simulink library "Ampere_Library"  (R2022b)
settings: Solver=FixedStepDiscrete  StartTime=0  StopTime=10.0  RelTol=1e-3  EnableMultiTasking=on
undefined symbols (not defined in the file or in its folder): A_INST_double, Dem_EventStatusType, ECU_AMBIENT_TEMPERATURE, SET_ECU_AMBIENT_TEMPERATURE, SlDemoSign, Std_ReturnType
libraries: simulink x13
(part 5 of 10)

== system Ampere_Library/User_Defined_Libraries/Signal_Routing ==
  note: Specific
  note: Invalid Values
  note: Signal Routing
  note: Obsolete
  A_DataTypeDuplicate : Subsystem  Tag=[LIB]  mask(A_DataTypeDuplicate){NoIn=3}
      mask prompts: NoIn "No Of Inputs"
      mask help:
      | ****************************************************************************
      | DO NOT USE THIS BLOCK ANYMORE.
      | Use the native "Same DT" block in the section MBD_Base_Blocks / Simulink / Signal_Attributes
      |
      | ****************************************************************************
      |
      | This block forces all inputs to have the exact same data type. The user shall set the number of the inputs in the mask parameter
      mask init:
      | % This code add/delete inports and matching lines to connect to the mux
      | % block.
      | 
      | % Number of inputs to have
      | f = str2num(get_param(gcb, 'NoIn'));
      | % Get all existing inports
      | d1 = find_system(gcb,'LookUnderMasks','all','Followlinks','on','BlockType','Inport');
      | 
      | % Update the mux block
      | set_param([gcb '/Mux'],'Inputs',num2str(f));
      | 
      | % Update content if new value different from number of existing inports
      | if f ~= length(d1)
      |     % Delete all existing inports and matching lines
      |     for i = 1:length(d1)
      |         hanblk = get_param(d1{i},'handle');
      |         blkDet = get(hanblk);
      |         pos = blkDet.PortConnectivity(1).Position;
      |         delete_line(gcb,pos);
      |         delete_block(d1{i});
      |     end
      |     
      |     % Add new ports and lintes
      |     for i = 1:f
      |         b = i*50;
      |         a = 150;
      |         append = num2str(i);
      |         append = strcat('/In',append);
      |     	PortName = strcat(gcb,append);
      |         add_block('built-in/Inport',PortName,'Position',[a-60 b-5 a-40 b+8],'FontName','Arial','FontSize',12);
      |         set_param(PortName,'ShowName','On')
      |         set_param(PortName,'Backgroundcolor','green');
      |         new_line = add_line(gcb,['In' num2str(i) '/1'],['Mux/' num2str(i)],'Autorouting','On');
      |         set(new_line,'FontName','Arial');
      |         set(new_line,'FontSize','12');
      |     end
      | end
      settings: AttributesFormatString="%<MaskType>  \\n No Of Inputs = %<NoIn>"
      mask Display:
      | %% Display info on the icon
      | fprintf('Same\nDT')
  A_DefaultValueSwitch : Subsystem  Tag=[LIB]  mask(A_DefaultValueSwitch){DefaultValue=15.1, InvalidValue=2.1, tolerance=double tol - eps('double'), user_tol=0, SaturateOnOverflow=off}
      mask prompts: DefaultValue "Default Value"; InvalidValue "Invalid Value"; tolerance "Tolerance for Invalid Value"; user_tol "User Defined Tolerance"; SaturateOnOverflow "Saturate on integer overflow"
      mask help:
      | This block outputs default value, in case of a invalid input. Otherwise output follows input.
      |
      | When parameter 'Invalid Value' and the input "U" is equal, then the output "Y" is equal to the 'Default Value' parameter. Otherwise the output "Y" is equal to the input "U".
      mask init:
      | %% Compute Tolerance
      | switch tolerance
      |     case 1
      |         tol = eps('double');
      |     case 2
      |         tol = eps('single');
      |     case 3
      |         tol = 0;
      |     case 4
      |         tol = user_tol;
      | end
      | 
      | %% Create the infos to display below the block depending of the Mask Options
      | % Always display MaskType
      | Attrib = '%<MaskType>';
      | % Conditionnally adding Tolerance
      | if strcmp(get_param(gcb,'tolerance'),'User Defined tol')
      |     Attrib = [Attrib '\nTol = %<user_tol>'];
      | end
      | % Conditionnally adding Sat
      | if strcmp(get_param(gcb,'SaturateOnOverflow'),'on')
      |     Attrib = [Attrib '\nSAT = on'];
      | end
      | % Update the display
      | set_param(gcb,'AttributesFormatString',Attrib);
      settings: AttributesFormatString=%<MaskType>
      mask TypeOptions tolerance: double tol - eps('double') | single tol - eps('single') | Absolute Zero tol | User Defined tol
      mask Callback tolerance:
      | %% Make visible or not the Tolerance (update 2nd element of MaskVisibilities)
      | MaskVisibilities = get_param(gcb,'MaskVisibilities');
      | if strcmp(get_param(gcb,'tolerance'),'User Defined tol')
      |     MaskVisibilities{4} = 'on';
      | else
      |     MaskVisibilities{4} = 'off';
      | end
      | set_param(gcb,'MaskVisibilities',MaskVisibilities);
      mask TypeOptions SaturateOnOverflow: Add/SaturateOnIntegerOverflow | Add1/SaturateOnIntegerOverflow | Switch2/SaturateOnIntegerOverflow
      mask Display:
      | %% Display info on the icon
      | fprintf('Default Val = %s\nInvalid Val = %s', get_param(gcb,'DefaultValue'),get_param(gcb,'InvalidValue'));
  A_ExtDefaultValueSw : Subsystem  Tag=[LIB]  mask(A_ExtDefaultValueSw){InvalidValue=0, tolerance=Absolute Zero tol, user_tol=2.5, SATonIntegerOverflow=off}
      mask prompts: InvalidValue "Invalid Value"; tolerance "Tolerance for Invalid Value"; user_tol "User Defined Tolerance"; SATonIntegerOverflow "Saturate on integer overflow"
      mask help:
      | When parameter 'Invalid Value' and input "Inp2" are equal then, the output "Y"  is equal to the input "Inp1". Otherwise the output "Y" is equal to the input "In2".
      | Note:
      | 1) If tolerance value is given for double/single data type, then the parameter "Invalid value" should be given within the range as given below
      | MAX value = ('double/single') MAX-Tolerance
      | MIN value = ('double/single') MIN+Tolerance
      mask init:
      | %% Compute Tolerance
      | switch tolerance
      |     case 1
      |         tol = eps('double');
      |     case 2
      |         tol = eps('single');
      |     case 3
      |         tol = 0;
      |     case 4
      |         tol = user_tol;
      | end
      | 
      | %% Create the infos to display below the block depending of the Mask Options
      | % Always display MaskType
      | Attrib = '%<MaskType>\nInvalidVal = %<InvalidValue>';
      | % Conditionnally adding Tolerance
      | if strcmp(get_param(gcb,'tolerance'),'User Defined tol')
      |     Attrib = [Attrib '\nTol = %<user_tol>'];
      | end
      | % Conditionnally adding Sat
      | if strcmp(get_param(gcb,'SATonIntegerOverflow'),'on')
      |     Attrib = [Attrib '\nSAT = on'];
      | end
      | % Update the display
      | set_param(gcb,'AttributesFormatString',Attrib);
      settings: AttributesFormatString=%<MaskType>\nInvalidVal = %<InvalidValue>
      mask TypeOptions tolerance: double tol - eps('double') | single tol - eps('single') | Absolute Zero tol | User Defined tol
      mask Callback tolerance:
      | %% Make visible or not the Tolerance (update 3nd element of MaskVisibilities)
      | MaskVisibilities = get_param(gcb,'MaskVisibilities');
      | if strcmp(get_param(gcb,'tolerance'),'User Defined tol')
      |     MaskVisibilities{3} = 'on';
      | else
      |     MaskVisibilities{3} = 'off';
      | end
      | set_param(gcb,'MaskVisibilities',MaskVisibilities);
      mask TypeOptions SATonIntegerOverflow: Switch2/SaturateOnIntegerOverflow | Add/SaturateOnIntegerOverflow | Add1/SaturateOnIntegerOverflow
  A_ResolutionBlock : Subsystem  Tag=[LIB]  mask(A_ResolutionBlock){Resolution=1, SaturateOnOverflow=off, prod_OutDataTypeStr=double}
      mask prompts: Resolution "Signal resolution resizing"; SaturateOnOverflow "Saturate on integer overflow"; prod_OutDataTypeStr "Simulink:blkprm_prompts:OUTPUT_UNIFIEDDATATYPE"
      mask help:
      | This block converts input signal 'U' value into the value 'Y', with resolution specified by 'Signal resolution resizing' mask parameter.
      |
      | Conversion is done using following formula:
      |
      | Y = [ROUND ( U / Resolution )] * Resolution
      |
      | Note:
      | 1.  Input (U) Datatype of the block must be "DOUBLE".
      | 2. Output data type of the block has to be chosen by the user through "Output data type" mask parameter.
      mask init:
      | %% Internal Parameters
      | RF0 = 0;
      | RF1 = 1;
      | RF05 = 0.5;
      settings: AttributesFormatString=%<MaskType>
      mask TypeOptions SaturateOnOverflow: Product1/SaturateOnIntegerOverflow
      mask Callback SaturateOnOverflow:
      | %% Create the infos to display below the block depending of the Mask Options
      | % Always display MaskType
      | Attrib = '%<MaskType>';
      | % Conditionnally adding Sat
      | if strcmp(get_param(gcb,'SaturateOnOverflow'),'on')
      |     Attrib = [Attrib '\nSAT = on'];
      | end
      | % Update the display
      | set_param(gcb,'AttributesFormatString',Attrib);
      mask TypeOptions prod_OutDataTypeStr: Product1/OutDataTypeStr
      mask DialogControl prod_OutDataTypeStr Prompt: Output data type:
      mask Display:
      | %% Display info on the icon
      | fprintf('Resol :\n%s', get_param(gcb,'Resolution'));
  A_SlopeSwitch2Inputs : Subsystem  Tag=[LIB]  mask(A_SlopeSwitch2Inputs){st=0.1, SaturateOnIntegerOverflow=off}
      mask prompts: st "Sample Time used for calculation, should not be inherited (-1)."; SaturateOnIntegerOverflow "Simulink:blkprm_prompts:AllBlksSaturate"
      mask help:
      | This block is a Multi-Port Slope Switch.
      | Depending on the value of input Switch_Cmd (zero-based), the block outputs the corresponding input signal.
      | For Switch_Cmd = 0, Outis Inp0, for Switch_Cmd = 1, Out is Inp1, and so on...
      |
      | Nevertheless, for each switch between two input signals, a slope is activated from the first input signal to the second input signal.
      | The value of this slope is given by Pos_Slope if the input signal to reach is over the initial input signal and by Neg_Slope if the input signal to reach is under.
      | Pos_Slope and Neg_Slope are respectively the positive and negative slope parameters per second.
      |
      | The output Slope_On indicates if a transition is active (Slope_On at true) or not (Slope_On at false).
      |
      | In order to avoid the overflow, the maximum/ minimun range for the inputs Pos_Slope and Neg_Slope shall be choosen as:
      | max range(Pos_Slope) = ( max range(data type(In))- max(In))
      | min range(Neg_Slope) = ( min range(data type(Input)) - min(Input))
      |
      | Note:
      | 1. Data type for the outport "Out" will be same as "Inp0" or "Inp1" (Inp0 and Inp1 should be same data type)
      | 2. Data type for the outport "Slope_On" is always "boolean".
      mask init:
      | %% Internal Parameters
      | InitDelay = 0;
      | InitOut = 0;
      settings: AttributesFormatString=%<MaskType>
      mask TypeOptions SaturateOnIntegerOverflow: Multiport_Switch/SaturateOnIntegerOverflow | Slope_On_Block/Product/SaturateOnIntegerOverflow | Slope_On_Block/Product1/SaturateOnIntegerOverflow | Slope_On_Block/Sum/SaturateOnIntegerOverflow | Slope_On_Block/Sum1/SaturateOnIntegerOverflow | Slope_On_Block/Switch1/SaturateOnIntegerOverflow | Slope_On_Block/Switch2/SaturateOnIntegerOverflow | Slope_On_Block/Switch3/SaturateOnIntegerOverflow | Switch2/SaturateOnIntegerOverflow
      mask Callback SaturateOnIntegerOverflow:
      | %% Create the infos to display below the block depending of the Mask Options
      | % Always display MaskType
      | Attrib = '%<MaskType>';
      | % Conditionnally adding Sat
      | if strcmp(get_param(gcb,'SaturateOnIntegerOverflow'),'on')
      |     Attrib = [Attrib '\nSAT = on'];
      | end
      | % Update the display
      | set_param(gcb,'AttributesFormatString',Attrib);
      mask DialogControl SaturateOnIntegerOverflow Prompt: Saturate on integer overflow
      mask Display:
      | %% Display info on the icon
      | color('blue')
      | fprintf('Slope switch\n\n2 Inputs')
  A_TwoInDefltValSwitch : Subsystem  Tag=[LIB]  mask(A_TwoInDefltValSwitch){DefaultValue=15.1, InvalidValue=2.1, tolerance=double tol - eps('double'), user_tol=2.5, SATOnIntegerOverflow=off}
      mask prompts: DefaultValue "Default Value"; InvalidValue "Invalid Value"; tolerance "Tolerance for Invalid Value"; user_tol "User Defined Tolerance"; SATOnIntegerOverflow "Saturate on integer overflow"
      mask help: Compare the input2 'U2' with the invalid value ,if it is equal then the output 'Y' is Default value,otherwise the output is as same as input1 'U1'.
      mask init:
      | %% Compute Tolerance
      | switch tolerance
      |     case 1
      |         tol = eps('double');
      |     case 2
      |         tol = eps('single');
      |     case 3
      |         tol = 0;
      |     case 4
      |         tol = user_tol;
      | end
      | 
      | %% Create the infos to display below the block depending of the Mask Options
      | % Always display MaskType
      | Attrib = '%<MaskType>';
      | % Conditionnally adding Tolerance
      | if strcmp(get_param(gcb,'tolerance'),'User Defined tol')
      |     Attrib = [Attrib '\nTol = %<user_tol>'];
      | end
      | % Conditionnally adding Sat
      | if strcmp(get_param(gcb,'SATOnIntegerOverflow'),'on')
      |     Attrib = [Attrib '\nSAT = on'];
      | end
      | % Update the display
      | set_param(gcb,'AttributesFormatString',Attrib);
      settings: AttributesFormatString=%<MaskType>
      mask TypeOptions tolerance: double tol - eps('double') | single tol - eps('single') | Absolute Zero tol | User Defined tol
      mask Callback tolerance:
      | %% Make visible or not the Tolerance (update 2nd element of MaskVisibilities)
      | MaskVisibilities = get_param(gcb,'MaskVisibilities');
      | if strcmp(get_param(gcb,'tolerance'),'User Defined tol')
      |     MaskVisibilities{4} = 'on';
      | else
      |     MaskVisibilities{4} = 'off';
      | end
      | set_param(gcb,'MaskVisibilities',MaskVisibilities);
      mask TypeOptions SATOnIntegerOverflow: Switch2/SaturateOnIntegerOverflow | Add/SaturateOnIntegerOverflow | Add1/SaturateOnIntegerOverflow
      mask Display:
      | %% Display info on the icon
      | fprintf('Default Val = %s\nInvalid Val = %s', get_param(gcb,'DefaultValue'), get_param(gcb,'InvalidValue'));
  A_demux_fc : Subsystem  Tag=[LIB]  Description=This block is let for backwards compatibility. Function-call generator blocks are forbiddenby LB001 rule. Users shall modify their models if this block is used.  mask(A_demux_fc){}
      mask help:
      | ****************************************************************************
      | DO NOT USE THIS BLOCK ANYMORE.
      | This block is let for backwards compatibility. Function-call generator blocks are forbiddenby LB001 rule. Users shall modify their models if this block is used
      | ****************************************************************************
      |
      | A_demux_fc block shall be use before demuxing function call signal.
      settings: AttributesFormatString=%<MaskType>  RTWSystemCode=Inline

== system Ampere_Library/User_Defined_Libraries/Sources ==
  note: Sources
  A_ClockGen : Subsystem  Tag=[LIB]  mask(A_ClockGen){st=0.1, SaturateOnOverflow=off, const_OutDataTypeStr=double}
      mask prompts: st "Sample time is used in calculation, should not be inherited (-1)"; SaturateOnOverflow "Saturate on integer overflow"; const_OutDataTypeStr "Sample time Datatype"
      mask help:
      | This block outputs the simulation time, when it is kept inside the time based subsystem. The parameter "sample time" should be explicitly mentioned.
      | Inherit value '-1' is not allowed.
      |
      | Note: Datatype of the given Sample time has to be chosen by the user through "Sample time Datatype" mask parameter.
      mask init:
      | %% Internal Parameter
      | InitClock = 0;
      | 
      | %% Check Sample Time
      | if st < 0
      |     errordlg(['Error : Do not use inherited sample time -1 in ',gcb]);
      | end
      settings: AttributesFormatString=|
      | %<MaskType>
      | Sample Time = %<st>
      mask TypeOptions SaturateOnOverflow: Sum1/SaturateOnIntegerOverflow
      mask Callback SaturateOnOverflow:
      | % Display the SaturateOnOverflow parameter only when 'on'
      | if strcmp(get_param(gcb,'SaturateOnOverflow'),'on')
      |     set_param(gcb, 'AttributesFormatString', sprintf('%%<MaskType>\nSample Time = %%<st> \nSAT = on'));
      | else
      |     set_param(gcb, 'AttributesFormatString', sprintf('%%<MaskType>\nSample Time = %%<st> \n'));
      | end
      mask TypeOptions const_OutDataTypeStr: st/OutDataTypeStr
      mask Display:
      | %% Display info on the icon
      | fprintf('Digital\nclock');
  A_DownEdge_Event : Subsystem  Tag=[LIB]  mask(A_DownEdge_Event){sample_time=0.01, event_time=0.1, InternalDT=double}
      mask prompts: sample_time "Sample time for calculations"; event_time "Event production time"; InternalDT "Internal Calculations Data Type"
      mask help:
      | Down edge event  : Every Event_time
      |
      | The block produces a Down Edge Boolean output every period of time defined by:
      | Event production time: period of time between two Down Edge events.
      |
      | * This block shall not be used inside triggered/enabled subsystem
      mask init:
      | %% Check for Internal Calculations Data Type 
      | if strcmp(get_param(gcb, 'InternalDT'), 'double')
      |     imm_clear = double(0);
      |     imm = double(0.0001);
      |     sample_time = double(sample_time);
      |     event_time = double(event_time);
      | else
      |     imm_clear = single(0);
      |     imm = single(0.0001);
      |     sample_time = single(sample_time);
      |     event_time = single(event_time);
      | end
      settings: AttributesFormatString=|
      | %<MaskType>
      | Internal DT = %<InternalDT>
      mask Display:
      | %% Display info on the icon
      | fprintf('Sample Time = %s\nEvent Time = %s', get_param(gcb,'sample_time'),get_param(gcb,'event_time'));
  A_EnumConstant : Subsystem  Tag=[LIB]  mask{OutDataTypeStr=Enum: SlDemoSign, EnumVal=Positive}
      mask prompts: OutDataTypeStr "Output data type"; EnumVal "Value"
      mask help: This block is customized to display an enumerated value in a more compact way and avoid giant blocks that degrade the readibility.
      mask init:
      | %% Retrieve the enum name and its value in the mask
      | Type = regexprep(strrep(get(gcbh,'OutDataTypeStr'),' ',''),'Enum:','');
      | Value = strtrim(get(gcbh,'EnumVal'));
      | 
      | %% Compute the enumerated value to put in the constant block
      | Ecst = eval([Type  '.'  Value]);
      settings: AttributesFormatString=Enum: SlDemoSign
      mask Callback OutDataTypeStr:
      | %% Get the enum name
      | Type = get(gcbh,'OutDataTypeStr');
      | 
      | %% Get its enumeration values as a char array to then create the new value
      | % of MaskStyles properties to update the popupmenu in the mask
      | ListVal = char(string(enumeration(regexprep(strrep(Type,' ',''),'Enum:',''))));
      | NewList = [];
      | for i = 1:size(ListVal,1)
      |     NewList = [NewList ListVal(i,:) '|'];
      | end
      | NewList(end) = [];
      | 
      | %% Update MaskStyles with the new values for the popupmenu
      | MaskStyles = get(gcbh,'MaskStyles');
      | MaskStyles{2} = ['popup(' NewList ')'];
      | set(gcbh,'MaskStyles',MaskStyles);
      | 
      | %% Update display below the block
      | set(gcbh,'AttributesFormatString',get(gcbh,'OutDataTypeStr'));
      mask TypeOptions EnumVal: Positive | Zero     | Negative
      mask Display:
      | %% Display the enum below the block and the value on the subsystem
      | fprintf('%s',strtrim(get(gcbh,'EnumVal')));

== system Ampere_Library/User_Defined_Libraries/Timers_and_Counters ==
  note: Timers
  note: Counters
  note: Turn On/Off Delays
  note: Timers & Counters
  A_COUNTER : Subsystem  Tag=[LIB]  mask(A_COUNTER){mMAX=1byte, SaturateOnOverflow=off}
      mask prompts: mMAX "Max. count range :"; SaturateOnOverflow "Saturate on integer overflow"
      mask help:
      | When the input of the block ("start_flag") gets the value 1 (True), the output value ("count_value") will be incremented at each simulation step until reaching the maximum value fixed by user and then, maintain the limit value.
      |
      | When the input of the block ("start_flag") gets the value 0 (False), the output value ("count_value") will be set to '0'
      |
      |
      | Note
      | The input of the block shall be a Boolean
      mask init:
      | %% Internal Parameters
      | IncrVal = 1;
      | ClrVal = 0;
      | IC_zero = 0;
      | 
      | %% Compute the limit value depending of the number of bytes
      | mMAX = get_param(gcb,'mMAX');
      | nbByte = str2double(mMAX(1)); % first element is either 1/2/4
      | MavVal = 2^(nbByte * 8 ) - 1;
      | 
      | if nbByte == 1
      |     limit_value = uint8(MavVal);
      | elseif nbByte == 2
      |     limit_value = uint16(MavVal);
      | else % nbByte == 4
      |     limit_value = uint32(MavVal);
      | end
      settings: AttributesFormatString=%<MaskType>
      mask TypeOptions mMAX: 1byte | 2byte | 4byte
      mask TypeOptions SaturateOnOverflow: Min/SaturateOnIntegerOverflow | Sum1/SaturateOnIntegerOverflow | Switch1/SaturateOnIntegerOverflow
      mask Callback SaturateOnOverflow:
      | %% Create the info to display below the block
      | Attrib = '%<MaskType>';
      | % Conditionnally display the SaturateOnOverflow parameter
      | if strcmp(get_param(gcb,'SaturateOnOverflow'),'on')
      |     Attrib = [Attrib '\nSAT = on'];
      | end
      | set_param(gcb, 'AttributesFormatString', Attrib);
      mask Display:
      | %% Display info on the icon
      | text(.5,.9,get_param(gcb,'mMAX'),'horizontalAlignment','center')
  A_Counter_Hold : Subsystem  Tag=[LIB]  mask(A_Counter_Hold){mMAX=2byte}
      mask prompts: mMAX "Max. count range :"
      mask help:
      | When the input of the block ("start_flag") gets the value 1 (True),
      | the output value ("count_value") will be incremented at each
      | simulation step until reaching the maximum value fixed by user
      | and then, keeps this value.
      |
      | When the input of the block ("start_flag") gets the value 0 (False), the output value ("count_value") is maintained (hold)
      |
      | When the input of the block ("clear_flag") gets the value 1(TRUE), the output value ("count_value") will be set to 0(reset)
      |
      | When the input of the block ("clear_flag") gets the value 0(FALSE), the output value ("count_value") depends on the input value ("start_flag")
      mask init:
      | %% Internal Parameters
      | SetVal = 1;
      | ClrVal = 0;
      | HoldVal = 0;
      | count_hold_init = 0;
      | 
      | %% Compute the limit value depending of the number of bytes
      | mMAX = get_param(gcb,'mMAX');
      | nbByte = str2double(mMAX(1)); % first element is either 1/2/4
      | MavVal = 2^(nbByte * 8 ) - 1;
      | if nbByte == 1
      |     limit_value = uint8(MavVal);
      | elseif nbByte == 2
      |     limit_value = uint16(MavVal);
      | else % nbByte == 4
      |     limit_value = uint32(MavVal);
      | end
      settings: AttributesFormatString=%<MaskType>
      mask TypeOptions mMAX: 1byte | 2byte | 4byte
      mask Display:
      | %% Display info on the icon
      | text(.5,.9,get_param(gcb,'mMAX'),'horizontalAlignment','center')
  A_IncAndDecCounter : Subsystem  Tag=[LIB]  mask(A_IncAndDecCounter){SaturateOnOverflow=off}
      mask prompts: SaturateOnOverflow "Saturate on integer overflow"
      mask help:
      | Initially the value of "Init_Counter" is set in the "Counter_Out" as initial value. If the "Inc_Counter" is true,
      | "Counter_Out" increases with the value of the "Counter_ Step". If the "Dec_Counter" is true and "Inc_Counter" is false,
      | the "Counter_Out" decreases with the value of the "Counter_ Step".
      |
      | The "Counter_Out" stops increasing or decreasing when it reaches to "Max_Counter" and " Min_Counter".
      | If the "Reset_Counter" is true, "Counter_Out" is reset to the value zero.
      |
      | Note:
      | 1. Inc_Counter, Dec_Counter and Reset_Counter inputs shall always be a boolean input and all other inputs shall be of same data type.
      |
      | 2. Output Data type shall be same as non-boolean input types.
      mask init:
      | %% Internal Parameters
      | Cons_Zero = uint8(0);
      | Cons_Zero_BP = uint8(0);
      | Cons_One = uint8(1);
      | Cons_Two = uint8(2);
      | Cons_Three = uint8(3);
      settings: AttributesFormatString=%<MaskType>
      mask TypeOptions SaturateOnOverflow: Add1/SaturateOnIntegerOverflow | Add2/SaturateOnIntegerOverflow | MinMax/SaturateOnIntegerOverflow | MinMax1/SaturateOnIntegerOverflow | Multiport_Switch/SaturateOnIntegerOverflow | Switch/SaturateOnIntegerOverflow
      mask Callback SaturateOnOverflow:
      | %% Create the info to display below the block
      | Attrib = '%<MaskType>';
      | % Conditionnally display the SaturateOnOverflow parameter
      | if strcmp(get_param(gcb,'SaturateOnOverflow'),'on')
      |     Attrib = [Attrib '\nSAT = on'];
      | end
      | set_param(gcb, 'AttributesFormatString', Attrib);
      mask DialogControl MaskParameter Prompt: Parameters
  A_Timer_Conversion : Subsystem  Tag=[LIB]  mask(A_Timer_Conversion){SampleTimeCst=1, SaturateOnOverflow=off}
      mask prompts: SampleTimeCst "Sample time :"; SaturateOnOverflow "Saturate on integer overflow"
      mask help:
      | A_Timer_Conversion block is to adapt the Input signal according to the Sample time specified in the block mask.
      |
      | Note:
      | 1) If the sample time is zero, then input is passed without any conversion.
      | 2) Sample time value shall not be less than zero.
      |
      | CAREFUL:
      | This legacy block is known to cause unreachable decision coverage.
      | It is kept in this library for ascending compatibility of legacy models.
      mask init:
      | %% Internal Parameters
      | Cons_0 = 0;
      settings: AttributesFormatString=%<MaskType>\nSample Time = %<SampleTimeCst>
      mask TypeOptions SaturateOnOverflow: Divide/SaturateOnIntegerOverflow | Switch/SaturateOnIntegerOverflow
      mask Callback SaturateOnOverflow:
      | %% Create the info to display below the block
      | Attrib = '%<MaskType>\nSample Time = %<SampleTimeCst>';
      | % Conditionnally display the SaturateOnOverflow parameter
      | if strcmp(get_param(gcb,'SaturateOnOverflow'),'on')
      |     Attrib = [Attrib '\nSAT = on'];
      | end
      | set_param(gcb, 'AttributesFormatString', Attrib);
      mask DialogControl ParameterTabVar0 Prompt: Constant
  A_Timer_Dec_Order : Subsystem  Tag=[LIB]  mask(A_Timer_Dec_Order){timeoutinit=0, initinit=0, st=0.1, SampleDT=single, SaturateOnOverflow=off, prod_OutDataTypeStr=single}
      mask prompts: timeoutinit "Timeout output initialisation"; initinit "Init input initialisation"; st "Sample Time used for calculation, should not be inherited (-1)."; SampleDT "DataType for Sample Time"; SaturateOnOverflow "Saturate on integer overflow for Internal Blocks"; prod_OutDataTypeStr "Simulink:blkprm_prompts:OUTPUT_UNIFIEDDATATYPE"
      mask help:
      | When the input1 of the block ("Init") is rising to 1, the following will be happening
      |     1. The output "Timer" will be set with "Duration" Value and start Decrementing by SampleTime.
      |     2. The output ("Timeout") will be Rising to 1 (TRUE) after a Delay (Duration/SampleTime).
      |
      | When the input1 of the block ("Init") is falling to 0, the following will be happening
      |     1. Block will be reset to Initial State (delay_out = 0 and Timer =0)
      |
      | Note:
      | 1. The Block's output "TimeOut" shall always be boolean.
      | 2. The Block's output "Timer" data type has to be chosen by the user through "Output data type" mask parameter.
      |
      | WARNING: Please note that Total Delay  = (Duration/SampleTime).
      mask init:
      | %% Internal Parameters
      | Tim1Ini = 0;
      | 
      | %% Compute the Boosting_Factor and the DT for floating points vs integers
      | fix_flag = ~isempty(regexp(get(gcbh,'SampleDT'),'^single$|^double$','once'));
      | if fix_flag
      |     Boosting_Factor = 1000;
      |     Constant_DT = get(gcbh,'SampleDT');
      | else
      |     Boosting_Factor = 1;
      |     Constant_DT = 'uint8';
      | end
      settings: AttributesFormatString=%<MaskType>\nTimeout init = %<timeoutinit>\nInput init = %<initinit>\nSample Time = %<st>
      mask TypeOptions SaturateOnOverflow: Product2/SaturateOnIntegerOverflow | Product3/SaturateOnIntegerOverflow | Product4/SaturateOnIntegerOverflow | Sum/SaturateOnIntegerOverflow | Switch2/SaturateOnIntegerOverflow | Switch3/SaturateOnIntegerOverflow | Switch4/SaturateOnIntegerOverflow
      mask Callback SaturateOnOverflow:
      | %% Create the info to display below the block
      | Attrib = '%<MaskType>\nTimeout init = %<timeoutinit>\nInput init = %<initinit>\nSample Time = %<st>';
      | % Conditionnally display the SaturateOnOverflow parameter
      | if strcmp(get_param(gcb,'SaturateOnOverflow'),'on')
      |     Attrib = [Attrib '\nSAT = on'];
      | end
      | set_param(gcb, 'AttributesFormatString', Attrib);
      mask TypeOptions prod_OutDataTypeStr: Product2/OutDataTypeStr
      mask DialogControl prod_OutDataTypeStr Prompt: Output data type:
      mask Display:
      | %% Ploting all figures
      | plot(0.1+[0.1 0.15 0.15 0.2 0.2 0.25],[0.67 0.67 0.9 0.9 0.67 0.67]);
      | plot([0.45 0.6 0.6 0.7],[0.67 0.67 0.9 0.9])
      | plot([0.45 0.5 0.5 0.6 0.7],.1+[0.05 0.05 0.3 0.05 0.05])
  A_Timer_Ext_TimeSt : Subsystem  Tag=[LIB]  mask(A_Timer_Ext_TimeSt){timeoutinit=0, initinit=0, dtype=Integer, SaturateOnOverflow=off, prod_OutDataTypeStr=Inherit: Inherit via back propagation}
      mask prompts: timeoutinit "Timeout output initialisation"; initinit "Init input initialisation"; dtype "Datatype of Timestep Signal"; SaturateOnOverflow "Saturate on integer overflow"; prod_OutDataTypeStr "Simulink:blkprm_prompts:OUTPUT_UNIFIEDDATATYPE"
      mask help:
      | When the input2 of the block ("Init") is rising to 1, the following will be happening
      |     1. The output ("Timeout") will be Rising to 1 (TRUE) after a Delay (Duration/Timestep).
      |     2. The output "Timer" will be set with "Duration" Value and start Decrementing by TimeStep input.
      |     3.  When the input3 of the block ("Timestep") is falling to 0,  Block will be reset to Initial State (Timeout = 0 and Timer = 0)
      |
      | Initializations:
      | - Output initialization = beginning state of Output signal.
      | - Input initialization = Used to determine rising or falling edge at the first simulation step.
      |     0 - Block will detect Edge Rising at the first simulation step itself
      |     1 - Block will detect Edge Rising at the first simulation step
      |
      | Warning: Please note that TotalDelay = (Duration/Timestep)
      |
      | Note:
      | 1. Negative Values are not allowed as an inputs (Duration,Timestep) to the block
      | 2. The Block's inputs (Duration,Timestep) must have Same Datatype and it should be Zero, when there is a Rising Edge of input (Init)
      | 3. The Block's output "TimeOut" shall always be boolean.
      | 4. The Block's output "Timer" data type has to be chosen by the user through "Output data type" mask parameter.
      mask init:
      | %% Internal Parameters
      | Tim1Ini = 0;
      | 
      | %% Compute the Boosting_Factor and the DT for floating points vs integers
      | if dtype == 1
      |     Boosting_FLP = 1000;
      |     Constant_DT = 'single';
      | elseif dtype == 2
      |     Boosting_FLP = 1000;
      |     Constant_DT = 'double';
      | else
      |     Boosting_FLP = 1;
      |     Constant_DT = 'uint32';
      | end
      settings: AttributesFormatString=%<MaskType>\nInput init = %<initinit>\nOutput init = %<timeoutinit>
      mask TypeOptions dtype: Single | Double | Integer
      mask TypeOptions SaturateOnOverflow: Product/SaturateOnIntegerOverflow | Product1/SaturateOnIntegerOverflow | Product2/SaturateOnIntegerOverflow | Sum/SaturateOnIntegerOverflow | Switch2/SaturateOnIntegerOverflow | Switch3/SaturateOnIntegerOverflow | Switch4/SaturateOnIntegerOverflow
      mask Callback SaturateOnOverflow:
      | %% Create the info to display below the block
      | Attrib = '%<MaskType>\nInput init = %<initinit>\nOutput init = %<timeoutinit>';
      | % Conditionnally display the SaturateOnOverflow parameter
      | if strcmp(get_param(gcb,'SaturateOnOverflow'),'on')
      |     Attrib = [Attrib '\nSAT = on'];
      | end
      | set_param(gcb, 'AttributesFormatString', Attrib);
      mask TypeOptions prod_OutDataTypeStr: Product2/OutDataTypeStr
      mask DialogControl prod_OutDataTypeStr Prompt: Output data type:
      mask Display:
      | %% Ploting all figures
      | plot(0.1+[0.1 0.15 0.15 0.2 0.2 0.25],[0.67 0.67 0.9 0.9 0.67 0.67]);
      | plot([0.45 0.6 0.6 0.7],[0.67 0.67 0.9 0.9])
      | plot([0.45 0.5 0.5 0.6 0.7],.1+[0.05 0.05 0.3 0.05 0.05])
  A_Timer_Hold_Inc_Order : Subsystem  Tag=[LIB]  mask(A_Timer_Hold_Inc_Order){sample_time=0.001}
      mask prompts: sample_time "Clock :"
      mask help:
      | Timer with holder
      |
      | I/O
      |  start_flag
      |    1 : timer count up
      |    0 : timer hold
      |  clear_flag
      |    1 : timer clear
      |    0 : timer operates according to the value of the input 'start_flag'
      |  target_time
      |    Target time
      |
      |  alarm
      |    1 : timer_value >= target_time
      |    0 : timer_value < target_time
      |  timer_value
      |    Timer value(up count)
      |
      | Note:
      | The two inputs 'start_flag' and 'clear_flag' shall be Boolean
      | The input 'target_time' can be either double or single datatype
      | The dialog parameter Clock specifies the counting step:
      | timer_value=timer_value_old+Clock
      mask init:
      | %% Internal Parameters
      | Resol = 0.0001;
      | ClrVal = 0;
      | TimKill = 0;
      | sample_time_init = 0;
      | alarm_init = 0;
      | 
      | %% Convert sample time in numerical value
      | SampleTime = str2double(get_param(gcb,'sample_time'));
      settings: AttributesFormatString=|
      | %<MaskType>
      | Clock = %<sample_time>
      mask TypeOptions sample_time: 0.001 | 0.002 | 0.004 | 0.01 | 0.02 | 0.1
  A_Timer_Inc_Order : Subsystem  Tag=[LIB]  mask(A_Timer_Inc_Order){sample_time=0.02}
      mask prompts: sample_time "Clock :"
      mask help:
      | Timer
      |
      | I/O
      |  start_flag
      |    1 : timer count up
      |    0 : timer clear
      |  target_time
      |    Target time
      |
      |  alarm
      |    1 : timer_value >= target_time
      |    0 : timer_value < target_time
      |  timer_value
      |    Timer value(up count)
      |
      | Note:
      | The input 'start_flag' shall be a Boolean
      | The input 'target_time' can be either double or single
      | The dialog parameter Clock specifies the counting step:
      | (timer_value=timer_value_old+Clock)
      mask init:
      | %% Internal Parameters
      | ClrVal = 0;
      | Resol = 0.0001;
      | Init_val = 0;
      | 
      | %% Convert sample time in numerical value
      | SampleTime = str2double(get_param(gcb,'sample_time'));
      settings: AttributesFormatString=|
      | %<MaskType>
      | Clock = %<sample_time>
      mask TypeOptions sample_time: 0.001 | 0.002 | 0.004 | 0.01 | 0.02 | 0.1
  A_TurnOffDly_Ctr_Out : Subsystem  Tag=[LIB]  mask(A_TurnOffDly_Ctr_Out){Ts=single(0.1), SampleDT=single, SATOnIntegerOverflow=off, prod_OutDataTypeStr=Inherit: Inherit via back propagation}
      mask prompts: Ts "Sample Time used for calculation, should not be inherited (-1)."; SampleDT "DataType for Sample Time"; SATOnIntegerOverflow "Saturate on integer overflow"; prod_OutDataTypeStr "Simulink:blkprm_prompts:OUTPUT_UNIFIEDDATATYPE"
      mask help:
      | When the input1 of the block ("delay_flag") is falling to 0, the following will be happening
      |     1. The output "Ctr" will be set with "Dly" Value and start Decrementing by SampleTime.
      |     2. The output ("delay_out") will be falling to 0 (FALSE) after a Delay (Dly/SampleTime).
      |
      | When the input1 of the block ("delay_flag") is rising to 1, the following will be happening
      |     1. Block will be reset to Initial State (delay_out = 1 and Ctr =0)
      |
      | WARNING: Please note that Total Delay  = (Dly/SampleTime).
      |
      | NOTE:
      |     1.When fixed data types is used for input ("dly"), both the input ("dly") and sample time (Ts specified in mask) should have the same resolution.
      |     2.When fixed data types is used for input ("dly"), the sample time's data type in the mask should be set as "Uint8".
      |     3.The input "dly" shall be set such that it is a multiple of sample time "Ts". Eg. If "dly" is 1 then allowed sample time (Ts) are 0.1,0.2,0.02, etc.,
      |    4. Output "delay_out" will always be boolean.
      |    5. Output "ctr" data type has to be chosen by the user through "Output data type" mask parameter.
      mask init:
      | %% Internal Parameters
      | IniVal = 0;
      | 
      | %% Update Boosting factor and DT
      | fix_flag = ~isempty(regexp(get(gcbh,'SampleDT'),'^single$|^double$','once'));
      | if fix_flag
      |     Boosting_Factor = 1000;
      |     Constant_DT = get(gcbh,'SampleDT');
      | else
      |     Boosting_Factor = 1;
      |     Constant_DT = 'uint8';
      | end
      settings: AttributesFormatString=%<MaskType>\nSample Time = %<Ts>
      mask TypeOptions SATOnIntegerOverflow: Product/SaturateOnIntegerOverflow | Product1/SaturateOnIntegerOverflow | Product3/SaturateOnIntegerOverflow | Sum1/SaturateOnIntegerOverflow | Switch1/SaturateOnIntegerOverflow | Switch2/SaturateOnIntegerOverflow | Switch3/SaturateOnIntegerOverflow
      mask Callback SATOnIntegerOverflow:
      | %% Create the info to display below the block
      | Attrib = '%<MaskType>\nSample Time = %<Ts>';
      | % Conditionnally display the SaturateOnOverflow parameter
      | if strcmp(get_param(gcb,'SATOnIntegerOverflow'),'on')
      |     Attrib = [Attrib '\nSAT = on'];
      | end
      | set_param(gcb, 'AttributesFormatString', Attrib);
      mask TypeOptions prod_OutDataTypeStr: Product3/OutDataTypeStr
      mask DialogControl prod_OutDataTypeStr Prompt: Output data type:
      mask Display:
      | %% Plot the line dly_flag
      | plot((2.5+[0  1  1  2  2  4  4  7  7  9  9 11])/16,...
      | 	 [10 10 8  8 10 10  8  8  8  8 10 10]/18);
      | text(.45,.55,'dly_flag');
      | %% Plot the line ctr
      | plot((2.5+[0  1  1  2  2  4  4  7  7  9  9 11])/16,...
      | 	 [4  4  7  6  6  6  7  4  4  4  4  4]/18);
      | text(.6,.3,'ctr');
      | %% Plot the line dly_out
      | plot((2.5+[0  1  1  2  2  4  4  7  7  9  9 11])/16,...
      | 	 [3  3  3  3  3  3  3  3  1  1  3  3]/18);
      | text(.33,.1,'dly_out');
  A_TurnOffDly_Ext_TimeSt : Subsystem  Tag=[LIB]  mask(A_TurnOffDly_Ext_TimeSt){outINI=false, inINI=false, SaturateOnOverflow=off, prod_OutDataTypeStr=Inherit: Inherit via back propagation}
      mask prompts: outINI "Output initialization (false or true)"; inINI "Input initialization (false or true)"; SaturateOnOverflow "Saturate on integer overflow"; prod_OutDataTypeStr "Simulink:blkprm_prompts:OUTPUT_UNIFIEDDATATYPE"
      mask help:
      | When the input1 of the block ("signal") is falling to 0, the following will be happening
      |     1. The output "Ctr" will be set with "Dly" Value and start Decrementing by TimeStep.
      |     2. The output ("out") will be falling to 0 (FALSE) after a Delay (DelayTime/ TimeStep).
      |
      | When the input1 of the block ("signal") is rising to 1, the following will be happening
      |     1. Block will be reset to Initial State (out = 1 and Ctr =0)
      |
      | WARNING: Please note that Total Delay  = (DelayTime / TimeStep).
      | Initializations:
      | - Output initialization = beginning state of Output signal.
      |
      | - Input initialization = Used to determine falling edge at the first simulation step.
      |    1 - Block will detect Edge Falling at the first simulation step itself.
      |    0 - Block will not detect Edge Falling at the first simulation step.
      |
      |
      | Note:
      | 1. Negative Values are not allowed as inputs("Delaytime" and "Timestep") for the block
      | 2. Inputs (Delaytime,Timestep) must have Same Datatype
      | 3. Inputs (Delaytime,Timestep) should not be Zero value when there is a Falling Edge of input (Signal)
      | 4. Output "out" shall always be boolean.
      | 5. Output "ctr" data type has to be chosen by the user using "Output data type" mask parameter.
      mask init:
      | %% Internal Parameters
      | Tim1Ini = 0;
      | Cons_1 = 1;
      | Cons_0 = 0;
      | Boosting_FLP = 1000;
      | Boosting_FXP = 1;
      | 
      | %% Update parameter depending of input mask options
      | if inINI == 2 % case true
      |     initinit = true;
      | else
      |     initinit = false;
      | end
      | 
      | %% Update parameter and internal block depending of output mask option
      | if outINI == 2 % case true
      |     timeoutinit = true;
      |     set_param([gcb '/From7'],'gototag','InitOut');
      | else
      |     timeoutinit = false;
      |     set_param([gcb '/From7'],'gototag','InitOut_Cond');
      | end
      settings: AttributesFormatString=%<MaskType>\nInput init = %<inINI>\nOutput init = %<outINI>
      mask TypeOptions outINI: false | true
      mask TypeOptions inINI: false | true
      mask TypeOptions SaturateOnOverflow: DataTypeConversion2/SaturateOnIntegerOverflow | Product/SaturateOnIntegerOverflow | Product1/SaturateOnIntegerOverflow | Product3/SaturateOnIntegerOverflow | Subtract4/SaturateOnIntegerOverflow | Sum/SaturateOnIntegerOverflow | Switch2/SaturateOnIntegerOverflow | Switch4/SaturateOnIntegerOverflow
      mask Callback SaturateOnOverflow:
      | %% Create the info to display below the block
      | Attrib = '%<MaskType>\nInput init = %<inINI>\nOutput init = %<outINI>';
      | % Conditionnally display the SaturateOnOverflow parameter
      | if strcmp(get_param(gcb,'SaturateOnOverflow'),'on')
      |     Attrib = [Attrib '\nSAT = on'];
      | end
      | set_param(gcb, 'AttributesFormatString', Attrib);
      mask TypeOptions prod_OutDataTypeStr: Product3/OutDataTypeStr
      mask DialogControl prod_OutDataTypeStr Prompt: Output data type:
      mask Display:
      | %% Plot the line dly_flag
      | plot((3.5+[0  1  1  2  2  4  4  7  7  9  9 11])/18,...
      | 	 .2+[10 10 8  8 10 10  8  8  8  8 10 10]/18);
      | text(.45,.74,'dly_flag');
      | %% Plot the line ctr
      | plot((3.5+[0  1  1  2  2  4  4  7  7  9  9 11])/18,...
      | 	 .2+[4  4  7  6  6  6  7  4  4  4  4  4]/18);
      | text(.6,.5,'ctr');
      | %% Plot the line dly_out
      | plot((3.5+[0  1  1  2  2  4  4  7  7  9  9 11])/18,...
      | 	 .2+[3  3  3  3  3  3  3  3  1  1  3  3]/18);
      | text(.33,.30,'dly_out');
  A_TurnOnDly_Ctr_Out : Subsystem  Tag=[LIB]  mask(A_TurnOnDly_Ctr_Out){Ts=single(0.1), SampleDT=single, SaturateOnOverflow=off, prod_OutDataTypeStr=single}
      mask prompts: Ts "Sample Time used for calculation, should not be inherited (-1)."; SampleDT "DataType for Sample Time"; SaturateOnOverflow "Saturate on integer overflow"; prod_OutDataTypeStr "Simulink:blkprm_prompts:OUTPUT_UNIFIEDDATATYPE"
      mask help:
      | When the input1 of the block ("delay_flag") is rising to 1, the following will be happening
      |     1. The output "Ctr" will be set with "Dly" Value and start Decrementing by SampleTime.
      |     2. The output ("delay_out") will be Rising to 1 (TRUE) after a Delay (Dly/SampleTime).
      |
      | When the input1 of the block ("delay_flag") is falling to 0, the following will be happening
      |     1. Block will be reset to Initial State (delay_out = 0 and Ctr =0)
      |
      | WARNING: Please note that Total Delay  = (Dly/SampleTime).
      |
      | Note:
      |    1. The Block's output "delay_out" shall always be boolean.
      |    2. The Block's output "ctr" data type has to be chosen by the user through "Output data type" mask parameter.
      mask init:
      | %% Internal Parameters
      | IniVal = 0;
      | 
      | %% Update Boosting factor and DT
      | fix_flag = ~isempty(regexp(get(gcbh,'SampleDT'),'^single$|^double$','once'));
      | if fix_flag
      |     Boosting_Factor = 1000;
      |     Constant_DT = get(gcbh,'SampleDT');
      | else
      |     Boosting_Factor = 1;
      |     Constant_DT = 'uint8';
      | end
      settings: AttributesFormatString=%<MaskType>\nSample Time = %<Ts>
      mask TypeOptions SaturateOnOverflow: Product/SaturateOnIntegerOverflow | Product1/SaturateOnIntegerOverflow | Product2/SaturateOnIntegerOverflow | Sum1/SaturateOnIntegerOverflow | Switch1/SaturateOnIntegerOverflow | Switch2/SaturateOnIntegerOverflow | Switch3/SaturateOnIntegerOverflow
      mask Callback SaturateOnOverflow:
      | %% Create the info to display below the block
      | Attrib = '%<MaskType>\nSample Time = %<Ts>';
      | % Conditionnally display the SaturateOnOverflow parameter
      | if strcmp(get_param(gcb,'SaturateOnOverflow'),'on')
      |     Attrib = [Attrib '\nSAT = on'];
      | end
      | set_param(gcb, 'AttributesFormatString', Attrib);
      mask TypeOptions prod_OutDataTypeStr: Product2/OutDataTypeStr
      mask DialogControl prod_OutDataTypeStr Prompt: Output data type:
      mask Display:
      | %% Plot the line dly_flag
      | plot((2.5+[0  1  1  2  2  4  4  7  7  9  9 11])/16,...
      | 	 [8  8 10 10  8  8 10 10 10 10  8  8]/18);
      | text(.45,.51,'dly_flag');
      | %% Plot the line ctr
      | plot((2.5+[0  1  1  2  2  4  4  7  7  9  9 11])/16,...
      | 	 [4  4  7  6  4  4  7  4  4  4  4  4]/18);
      | text(.6,.3,'ctr');
      | %% Plot the line dly_out
      | plot((2.5+[0  1  1  2  2  4  4  7  7  9  9 11])/16,...
      | 	 [1  1  1  1  1  1  1  1  3  3  1  1]/18);
      | text(.33,.15,'dly_out');
  A_TurnOnDly_Ext_TimeSt : Subsystem  Tag=[LIB]  mask(A_TurnOnDly_Ext_TimeSt){timeoutinit=false, initinit=false, dtype=Single, SaturateOnOverflow=off}
      mask prompts: timeoutinit "Output initialization (false or true)"; initinit "Input initialization (false or true)"; dtype "Datatype of Timestep Signal"; SaturateOnOverflow "Saturate on integer overflow"
      mask help:
      | When the input2 of the block ("Signal") is rising to 1, the following will be happening
      |     1. The output ("Out") will be Rising to 1 (TRUE) after a Delay (Delaytime/Timestep).
      |
      | When the input3 of the block ("Timestep") is falling to 0, the following will be happening
      |     1. Block will be reset to Initial State (Out = 0)
      |
      | Initializations:
      | - Output initialization = beginning state of Output signal.
      | - Input initialization = Used to determine rising or falling edge at the first simulation step.
      |     0 - Block will detect Edge Rising at the first simulation step itself
      |     1 - Block will detect Edge Rising at the first simulation step
      |
      | Warning: Please note that TotalDelay = (Delaytime/Timestep)
      |
      | Note:
      | 1. Negative Values are not allowed as an inputs (Delaytime,Timestep) to the block
      | 2. The Block's inputs (Delaytime,Timestep) must have Same Datatype
      | 3. The Block's inputs (Delaytime,Timestep) should not be Zero value when there is a Rising Edge of input (Signal)
      mask init:
      | %% Internal Parameters
      | Tim1Ini = 0;
      | 
      | %% Update the Boosting factor and DT
      | if dtype == 1
      |     Boosting_FLP = 1000;
      |     set_param([gcb '/Elab_TimeStepSup/BOOSTING_FLP'],'OutDatatypestr','double');
      | elseif dtype == 2
      |     Boosting_FLP = 1000;
      |     set_param([gcb '/Elab_TimeStepSup/BOOSTING_FLP'],'OutDatatypestr','single');
      | else
      |     Boosting_FLP = 1;
      |     set_param([gcb '/Elab_TimeStepSup/BOOSTING_FLP'],'OutDatatypestr','uint8');
      | end
      | 
      | %% Variant choice
      | TimeOutInit = get_param(gcb,'timeoutinit');
      | variant_select = evalin('base',TimeOutInit);
      | if ~any(strcmp(TimeOutInit,{'1','true','0','false'}))
      |     fprintf(2,'Init values shall be booleans true/false for the block %s\n',gcb);
      | end
      | 
      | %% Set active variant
      | if isequal(variant_select,1)    
      |     set_param([gcb '/VariantInitOutput'],'OverrideUsingVariant','Variant1');
      | else
      |     set_param([gcb '/VariantInitOutput'],'OverrideUsingVariant','(default)');
      | end
      settings: AttributesFormatString=%<MaskType>\nInput init = %<initinit>\nOutput init = %<timeoutinit>
      mask TypeOptions dtype: Double | Single | Integer
      mask TypeOptions SaturateOnOverflow: Elab_TimeStepSup/Product/SaturateOnIntegerOverflow | Elab_TimeStepSup/Product1/SaturateOnIntegerOverflow | Elab_TimeStepSup/Sum/SaturateOnIntegerOverflow
      mask Callback SaturateOnOverflow:
      | %% Create the info to display below the block
      | Attrib = '%<MaskType>\nInput init = %<initinit>\nOutput init = %<timeoutinit>';
      | % Conditionnally display the SaturateOnOverflow parameter
      | if strcmp(get_param(gcb,'SaturateOnOverflow'),'on')
      |     Attrib = [Attrib '\nSAT = on'];
      | end
      | set_param(gcb, 'AttributesFormatString', Attrib);
      mask Display:
      | %% Ploting all figures
      | plot([3 3.5 3.5 4 4 5 5 7.5 7.5 8.5], [5 5 6 6 5 5 6 6 5 5]);
      | plot([3 6.5 6.5 7.5 7.5 8.5], [2 2 3 3 2 2]);
      | plot([3 4.5], [5 6]);
      | plot([3 4.5], [6 5]);
      | text(5,0.4, 'Duration');
      | plot([5 6.5], [1 1]);
      | plot([5.2 5 5.2], [0.8 1 1.2]);
      | plot([6.3 6.5 6.3], [0.8 1 1.2]);
      | plot([5 5],[4.7 1.3]);
      | plot([6.5 6.5],[1.8 1.3]);
      | plot([7.5 7.5],[4.7 3.7]);
      | plot([0], [0]);
      | plot([8], [7]);

== system Ampere_Library/Basic_Software_Operation/Diagnostic_Event_Manager/A_ReportDiagnosticTestResult ==
  note: Updated through mask callback
  note: Refer Mask Description of this Library block for detailed information.
  note: Block with high width as the function name length depends of the name in the mask.
  TestResult : Inport  OutDataTypeStr=boolean
      settings: AttributesFormatString=DT = %<OutDataTypeStr>
  DEM_EVENT_STATUS_F : Constant  Value=Dem_EventStatusType.DEM_EVENT_STATUS_PREFAILED
  DEM_EVENT_STATUS_P : Constant  Value=Dem_EventStatusType.DEM_EVENT_STATUS_PREPASSED
  DemSetEventStatusCall : FunctionCaller  FunctionPrototype=ERR = DEVICE2_SC_TO_GND3_setEventStatus(EventStatus)  InputArgumentSpecifications=Dem_EventStatusType(1)  OutputArgumentSpecifications=uint8(0)
  Switch1 : Switch  Criteria=u2 ~= 0  RndMeth=Zero  SaturateOnIntegerOverflow=off
  Terminator : Terminator
  wires:
  DEM_EVENT_STATUS_P/1 -> Switch1/3
  TestResult/1 -> Switch1/2
  DEM_EVENT_STATUS_F/1 -> Switch1/1
  Switch1/1 -> DemSetEventStatusCall/1
  DemSetEventStatusCall/1 -> Terminator/1
